simulink model "PhaseII_opalrt_NoProtection"  (Simulink 8.8)
settings: Solver=ode3  StartTime=0.0  StopTime=inf  FixedStep=Ts  RelTol=1e-5  EnableMultiTasking=on
PostLoadFcn:
  | %BESS ctrl
  | Kpf=0.005*3*12;
  | Kif=5*6;
  | 
  | Kpf1=0.005*3*12;
  | Kif1=5*6;
  | Kp_v=0.016*15*35;
  | Ki_v=12*25;
  | 
  | Kp_v1=0.016*15*35;
  | Ki_v1=12*25;
  | 
  | Vabc_B=12.47e3;
  | Vdc_ref=Vabc_B*2;
  | Kpwm=sqrt(2)*Vabc_B/Vdc_ref;
  | ZB=Vabc_B^2/1e6;
  | R=0.005*ZB;
  | Ibasefull=673/2*sqrt(2);
  | 
  | 
  | Ts_Control=1e-4;
  | ts=0.05;
  | delay=0.2;
  | offset=10e3;
  | t_plan=60;
  | t_monitor=.2;
  | t_mon=t_monitor;
  | scalingfactor=1;
  | x=0.5;
  | n=6;
  | %t_plan=1/15;
  | %t_monitor=10/900;
  | %t_mon=10/900;
  | 
  | %t_plan=1/5;
  | %t_monitor=10/300;
  | %t_mon=10/300;
  | %scalingfactor=1/300;
  | 
  | f0=60;
  | 
  | Pabc_B=1e6;
  | Iabc_B=Pabc_B*sqrt(2/3)/Vabc_B;  % pk value
  | Imax_1=2.5;
  | Ptrans_B=Pabc_B*200;
  | 
  | Vdc_ref=Vabc_B*2;
  | 
  | ZB=Vabc_B^2/Pabc_B;
  | L=0.1*ZB/2/pi/60;
  | R=0.1*ZB;
  | C=1/(4*pi^2*(2e3)^2*L);
  | 
  | LL=0.005*ZB/2/pi/60;
  | RR=0.005*ZB;
  | 
  | RC=0.02;
  | 
  | %%% Initial SOC %%%%
  | SOC_ini_BESS1=0.5;
  | ... (+223 lines)
InitFcn:
  | %BESS ctrl
  | Kpf=0.005*3*12;
  | Kif=5*6;
  | 
  | Kpf1=0.005*3*12;
  | Kif1=5*6;
  | Kp_v=0.016*15*35;
  | Ki_v=12*25;
  | 
  | Kp_v1=0.016*15*35;
  | Ki_v1=12*25;
  | 
  | Vabc_B=12.47e3;
  | Vdc_ref=Vabc_B*2;
  | Kpwm=sqrt(2)*Vabc_B/Vdc_ref;
  | ZB=Vabc_B^2/1e6;
  | R=0.005*ZB;
  | Ibasefull=673/2*sqrt(2);
  | 
  | 
  | Ts_Control=1e-4;
  | ts=0.05;
  | delay=0.2;
  | offset=10e3;
  | t_plan=60;
  | t_monitor=.2;
  | t_mon=t_monitor;
  | scalingfactor=1;
  | x=0.5;
  | n=6;
  | %t_plan=1/15;
  | %t_monitor=10/900;
  | %t_mon=10/900;
  | 
  | %t_plan=1/5;
  | %t_monitor=10/300;
  | %t_mon=10/300;
  | %scalingfactor=1/300;
  | 
  | f0=60;
  | 
  | Pabc_B=1e6;
  | Iabc_B=Pabc_B*sqrt(2/3)/Vabc_B;  % pk value
  | Imax_1=2.5;
  | Ptrans_B=Pabc_B*200;
  | 
  | Vdc_ref=Vabc_B*2;
  | 
  | ZB=Vabc_B^2/Pabc_B;
  | L=0.1*ZB/2/pi/60;
  | R=0.1*ZB;
  | C=1/(4*pi^2*(2e3)^2*L);
  | 
  | LL=0.005*ZB/2/pi/60;
  | RR=0.005*ZB;
  | 
  | RC=0.02;
  | 
  | %%% Initial SOC %%%%
  | SOC_ini_BESS1=0.5;
  | ... (+223 lines)
undefined symbols (not defined in the file): D1, Delta, DiscIntNeverNeededParam, Left, PG2ref, type, V
libraries: powerlib x220, powerlib_meascontrol x82, dspstat3 x54, dsparch4 x43, dspswit3 x24, simulink x19, simulink_extras x12, powerlib_extras x11, ssn_lib x7, artemis x6, rtlab x5, rtio_generic_dnp3 x5
(part 4 of 9)

== system PhaseII_opalrt_NoProtection/SM_System/PV Farm 2 MW1 ==
  Demux2 : Demux  Outputs=3
  Gain5 : Gain  Gain=Vdc_ref/2
  vsa : powerlib/Electrical Sources/Controlled Voltage Source  Initialize=on  Source_Type=AC  Amplitude=0  Phase=0  Frequency=0  Measurements=None
  vsb : powerlib/Electrical Sources/Controlled Voltage Source  Initialize=on  Source_Type=AC  Amplitude=0  Phase=0  Frequency=0  Measurements=None
  vsc : powerlib/Electrical Sources/Controlled Voltage Source  Initialize=on  Source_Type=AC  Amplitude=0  Phase=0  Frequency=0  Measurements=None
  A : PMIOPort  Tag=PMCPort  Port=1  Side=Right
  B : PMIOPort  Tag=PMCPort  Port=2  Side=Right
  C : PMIOPort  Tag=PMCPort  Port=3  Side=Right
  wires:
  Demux2/1 -> vsa/1
  Demux2/2 -> vsb/1
  Demux2/3 -> vsc/1
  [Vref_PV1] -> Gain5/1
  Gain5/1 -> Demux2/1
  connections:
  vsa/LConn1 -- vsc/LConn1 -- vsb/LConn1
  vsc/RConn1 -- C/RConn1
  B/RConn1 -- vsb/RConn1
  vsa/RConn1 -- A/RConn1

== system PhaseII_opalrt_NoProtection/SM_System/Subsystem ==
  In1 : Inport
  Fault : Subsystem
  Ground : powerlib/Elements/Ground  LConnTagsString=a
  Three-Phase Series RLC Branch5 : powerlib/Elements/Three-Phase Series RLC Branch  LConnTagsString=A|B|C  RConnTagsString=A|B|C  BranchType=RL  Resistance=1e-2  Inductance=1e-2  Capacitance=1e-4  Measurements=None
  a : PMIOPort  Port=1  Side=Left
  b : PMIOPort  Port=2  Side=Left
  c : PMIOPort  Port=3  Side=Left
  wires:
  In1/1 -> Fault/1(In7)
  connections:
  Ground/LConn1 -- Three-Phase Series RLC Branch5/LConn3 -- Three-Phase Series RLC Branch5/LConn2 -- Three-Phase Series RLC Branch5/LConn1
  Fault/RConn2 -- Three-Phase Series RLC Branch5/RConn2
  Fault/RConn3 -- Three-Phase Series RLC Branch5/RConn3
  Fault/RConn1 -- Three-Phase Series RLC Branch5/RConn1
  a/RConn1 -- Fault/LConn1
  b/RConn1 -- Fault/LConn2
  c/RConn1 -- Fault/LConn3

== system PhaseII_opalrt_NoProtection/SM_System/Subsystem1 ==
  In1 : Inport
  Fault : Subsystem
  Ground : powerlib/Elements/Ground  LConnTagsString=a
  Three-Phase Series RLC Branch5 : powerlib/Elements/Three-Phase Series RLC Branch  LConnTagsString=A|B|C  RConnTagsString=A|B|C  BranchType=RL  Resistance=1e-2  Inductance=1e-2  Capacitance=1e-4  Measurements=None
  a : PMIOPort  Port=1  Side=Left
  b : PMIOPort  Port=2  Side=Left
  c : PMIOPort  Port=3  Side=Left
  wires:
  In1/1 -> Fault/1(In7)
  connections:
  c/RConn1 -- Fault/LConn3
  b/RConn1 -- Fault/LConn2
  a/RConn1 -- Fault/LConn1
  Fault/RConn1 -- Three-Phase Series RLC Branch5/RConn1
  Fault/RConn3 -- Three-Phase Series RLC Branch5/RConn3
  Fault/RConn2 -- Three-Phase Series RLC Branch5/RConn2
  Three-Phase Series RLC Branch5/LConn1 -- Three-Phase Series RLC Branch5/LConn2 -- Three-Phase Series RLC Branch5/LConn3 -- Ground/LConn1

== system PhaseII_opalrt_NoProtection/SM_System/Subsystem2 ==
  In1 : Inport
  Fault : Subsystem
  Ground : powerlib/Elements/Ground  LConnTagsString=a
  Three-Phase Series RLC Branch5 : powerlib/Elements/Three-Phase Series RLC Branch  LConnTagsString=A|B|C  RConnTagsString=A|B|C  BranchType=RL  Resistance=1e-2  Inductance=1e-2  Capacitance=1e-4  Measurements=None
  a : PMIOPort  Port=1  Side=Left
  b : PMIOPort  Port=2  Side=Left
  c : PMIOPort  Port=3  Side=Left
  wires:
  In1/1 -> Fault/1(In7)
  connections:
  Ground/LConn1 -- Three-Phase Series RLC Branch5/LConn3 -- Three-Phase Series RLC Branch5/LConn2 -- Three-Phase Series RLC Branch5/LConn1
  Fault/RConn2 -- Three-Phase Series RLC Branch5/RConn2
  Fault/RConn3 -- Three-Phase Series RLC Branch5/RConn3
  Fault/RConn1 -- Three-Phase Series RLC Branch5/RConn1
  a/RConn1 -- Fault/LConn1
  b/RConn1 -- Fault/LConn2
  c/RConn1 -- Fault/LConn3

== system PhaseII_opalrt_NoProtection/SM_System/Subsystem3 ==
  In1 : Inport
  Fault : Subsystem
  Ground : powerlib/Elements/Ground  LConnTagsString=a
  Three-Phase Series RLC Branch5 : powerlib/Elements/Three-Phase Series RLC Branch  LConnTagsString=A|B|C  RConnTagsString=A|B|C  BranchType=RL  Resistance=1e-2  Inductance=1e-2  Capacitance=1e-4  Measurements=None
  a : PMIOPort  Port=1  Side=Left
  b : PMIOPort  Port=2  Side=Left
  c : PMIOPort  Port=3  Side=Left
  wires:
  In1/1 -> Fault/1(In7)
  connections:
  c/RConn1 -- Fault/LConn3
  b/RConn1 -- Fault/LConn2
  a/RConn1 -- Fault/LConn1
  Fault/RConn1 -- Three-Phase Series RLC Branch5/RConn1
  Fault/RConn3 -- Three-Phase Series RLC Branch5/RConn3
  Fault/RConn2 -- Three-Phase Series RLC Branch5/RConn2
  Three-Phase Series RLC Branch5/LConn1 -- Three-Phase Series RLC Branch5/LConn2 -- Three-Phase Series RLC Branch5/LConn3 -- Ground/LConn1

== system PhaseII_opalrt_NoProtection/SM_System/Subsystem4 ==
  In1 : Inport
  Fault : Subsystem
  Ground : powerlib/Elements/Ground  LConnTagsString=a
  Three-Phase Series RLC Branch5 : powerlib/Elements/Three-Phase Series RLC Branch  LConnTagsString=A|B|C  RConnTagsString=A|B|C  BranchType=RL  Resistance=1e-2  Inductance=1e-2  Capacitance=1e-4  Measurements=None
  a : PMIOPort  Port=1  Side=Left
  b : PMIOPort  Port=2  Side=Left
  c : PMIOPort  Port=3  Side=Left
  wires:
  In1/1 -> Fault/1(In7)
  connections:
  Ground/LConn1 -- Three-Phase Series RLC Branch5/LConn3 -- Three-Phase Series RLC Branch5/LConn1 -- Three-Phase Series RLC Branch5/LConn2
  Fault/RConn2 -- Three-Phase Series RLC Branch5/RConn2
  Fault/RConn3 -- Three-Phase Series RLC Branch5/RConn3
  Fault/RConn1 -- Three-Phase Series RLC Branch5/RConn1
  a/RConn1 -- Fault/LConn1
  b/RConn1 -- Fault/LConn2
  c/RConn1 -- Fault/LConn3

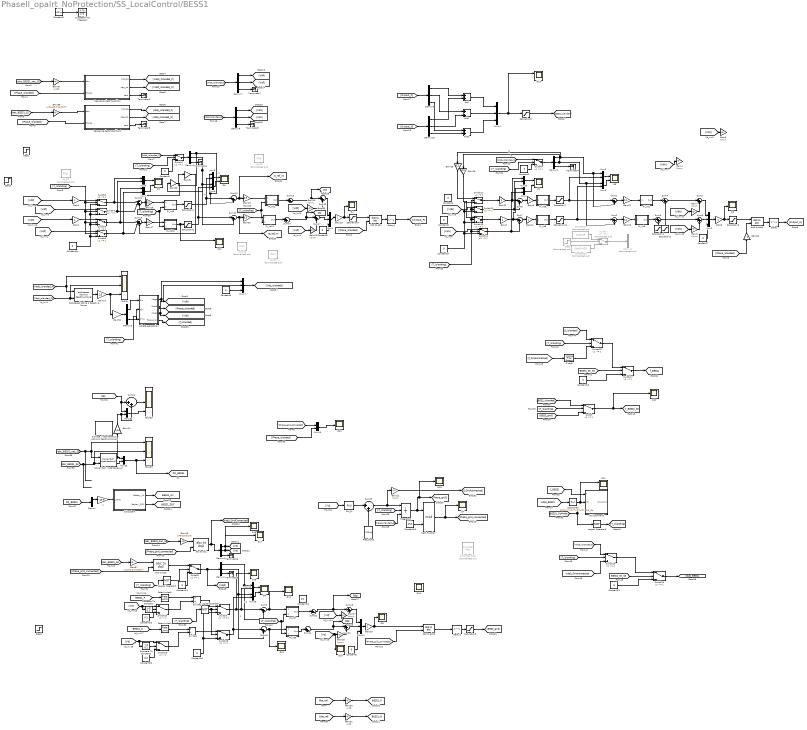
== system PhaseII_opalrt_NoProtection/SS_LocalControl/BESS1 ==
  "     1" : Gain  Gain=-1e-6
  2 kHz5 : dsparch4/Analog Filter Design  method=Butterworth  filttype=Lowpass  N=2  Wlo=2*pi*1  Whi=80  Rp=2  Rs=40
  2nd-Order Filter : powerlib_extras/Control  Blocks/2nd-Order Filter  Commented=on  FilterType=Lowpass  Fo=25  Zeta=0.707  Initialize=on  Vac_Init=[0 0 60]  Vdc_Init=377  PlotResponse=off  param1=[1 1000 0.5]
  3-phase  Instantaneous  Active & Reactive Power3 : powerlib_extras/Measurements/3-phase  Instantaneous  Active & Reactive Power
  Add : Sum
  Add1 : Sum
  Add2 : Sum
  Compare To Constant : simulink/Logic and Bit Operations/Compare To Constant  relop=>=  const=0.2  OutDataTypeStr=boolean
  Compare To Constant1 : simulink/Logic and Bit Operations/Compare To Constant  relop=>=  const=0.2  OutDataTypeStr=boolean
  Constant{1..2,4..11,13..14,17,21} (14 alike) : Constant  Value=0  SampleTime=-1
  Constant12 : Constant  Value=0.1  SampleTime=-1
  Constant15 : Constant  Value=2*pi
  Constant16 : Constant  Value=0.2  SampleTime=-1
  Constant18 : Constant  Commented=on  Value=[Kpf1 Kif1]  SampleTime=-1
  Constant19 : Constant  Commented=on  Value=[Kpf Kif]  SampleTime=-1
  Constant20 : Constant  Value=0.2  SampleTime=-1
  Constant3 : Constant  Value=120*pi
  D{1..2,5..6,9,15,22} (7 alike) : Scope  NumInputPorts=2
  D{3..4,7..8,10..14,16..20} (14 alike) : Scope
  D21 : Scope  NumInputPorts=3
  Delay : Delay  DelayLength=1  InitialCondition=0
  Delay1 : Delay  DelayLength=1  InitialCondition=0
  Delay2 : Delay  DelayLength=1  InitialCondition=0
  Demux : Demux  Outputs=2
  Demux1 : Demux  Commented=on  Outputs=2
  Demux{2,4..10} (8 alike) : Demux  Outputs=3
  Demux3 : Demux  Outputs=2
  Discrete-Time Integrator : DiscreteIntegrator  SampleTime=-1  ICPrevOutput=DiscIntNeverNeededParam  ICPrevScaledInput=DiscIntNeverNeededParam
  Divide1 : Product  Inputs=*/
  Divide2 : Product  Inputs=*/
  Freq_Const : Constant  Value=120*pi
  Gain{1..3,6,8,11,15,22,29} (9 alike) : Gain
  Gain{4..5,7,9..10,13,27..28} (8 alike) : Gain  Gain=Kpwm
  Gain12 : Gain  Gain=0.1
  Gain14 : Gain  Gain=2/3
  Gain{16..18,20} (4 alike) : Gain  Gain=0.5
  Gain19 : Gain  Gain=1/480/sqrt(2/3)
  Gain21 : Gain  Gain=1/2/pi
  Gain23 : Gain  Gain=0.1
  Gain24 : Gain  Gain=-1e-6
  Gain25 : Gain  Gain=0.2
  Gain26 : Gain  Gain=0.2
  Gain30 : Gain  Gain=-4.38
  Gain31 : Gain  Gain=-4.38
  Gain32 : Gain  Gain=0.228
  Gain33 : Gain  Gain=0.12
  Gain34 : Gain  Gain=0.12
  Gain36 : Gain  Gain=-1
  Gain37 : Gain  Gain=1/sqrt(2/3)/Ibasefull
  Gain38 : Gain  Gain=1/Ibasefull/sqrt(2/3)
  Gain57 : Gain  Gain=1/480
  ID&IQ : Scope  NumInputPorts=3
  ID&IQ1 : Scope  NumInputPorts=3
  ID&IQ2 : Scope  NumInputPorts=3
  Integrator1 : Integrator  ExternalReset=falling  InitialConditionSource=external  LimitOutput=on
  Logical Operator : Logic  Operator=NOT  Inputs=1  AllPortsSameDT=off  OutDataTypeStr=boolean
  Logical Operator1 : Logic  Operator=NOT  Inputs=1  AllPortsSameDT=off  OutDataTypeStr=boolean
  Logical Operator3 : Logic  Operator=NOT  AllPortsSameDT=off  OutDataTypeStr=boolean
  Math Function : Math  Operator=mod  SaturateOnIntegerOverflow=on
  Mux{1..2,11,14,17} (5 alike) : Mux  Inputs=3
  Mux{3..10,12..13,15..16,18} (13 alike) : Mux  Inputs=2
  PI_Vd1 : Subsystem
  PI_Vd10 : Subsystem
  PI_Vd11 : Subsystem
  PI_Vd2 : Subsystem
  PI_Vd3 : Subsystem
  PI_Vd5 : Subsystem
  PI_Vd6 : Subsystem
  PI_Vd7 : Subsystem
  PI_Vd8 : Subsystem
  PI_Vd9 : Subsystem
  PLL_PI : simulink/Continuous/PID Controller  Controller=PI  TimeDomain=Continuous-time  SampleTime=-1  IntegratorMethod=Forward Euler  FilterMethod=Forward Euler  Form=Parallel  UseFilter=on  ControllerParametersSource=internal  P=53*100  I=900*100  D=0  N=100  InitialConditionSource=internal  InitialConditionForIntegrator=0  InitialConditionForFilter=0  ExternalReset=none  ZeroCross=off  LimitOutput=on  UpperSaturationLimit=20  LowerSaturationLimit=-20  LinearizeAsGain=off  AntiWindupMode=clamping  Kb=1  TrackingMode=off  Kt=1  PParamMin=[]  PParamMax=[]  IParamMin=[]  IParamMax=[]  DParamMin=[]  DParamMax=[]  NParamMin=[]  NParamMax=[]  KbParamMin=[]  KbParamMax=[]  KtParamMin=[]  KtParamMax=[]  POutMin=[]  POutMax=[]  IOutMin=[]  IOutMax=[]  DOutMin=[]  DOutMax=[]  NOutMin=[]  NOutMax=[]  KbOutMin=[]  KbOutMax=[]  KtOutMin=[]  KtOutMax=[]  IntegratorOutMin=[]  IntegratorOutMax=[]  FilterOutMin=[]  FilterOutMax=[]  SumOutMin=[]  SumOutMax=[]  SumI1OutMin=[]  SumI1OutMax=[]  SumI2OutMin=[]  SumI2OutMax=[]  SumI3OutMin=[]  SumI3OutMax=[]  SumDOutMin=[]  SumDOutMax=[]  SaturationOutMin=[]  SaturationOutMax=[]  IntegratorContinuousStateAttributes=''  IntegratorStateMustResolveToSignalObject=off  IntegratorRTWStateStorageClass=Auto  FilterContinuousStateAttributes=''  FilterStateMustResolveToSignalObject=off  FilterRTWStateStorageClass=Auto  DifferentiatorICPrevScaledInput=0  DifferentiatorOutMin=[]  DifferentiatorOutMax=[]
  "Power (3ph, Instantaneous)" : powerlib_meascontrol/Measurements/Power (3ph, Instantaneous)
  Rate Limiter1 : RateLimiter  SampleTimeMode=inherited
  Rate Limiter2 : RateLimiter  SampleTimeMode=inherited
  SW Command : Subsystem
  Saturation1 : Saturate  UpperLimit=0.95  LowerLimit=-0.95
  Saturation10 : Saturate  UpperLimit=2  LowerLimit=-2  ZeroCross=off
  Saturation2 : Saturate  UpperLimit=0.95  LowerLimit=-0.95
  Saturation3 : Saturate  UpperLimit=1  LowerLimit=-1
  Saturation4 : Saturate  UpperLimit=4  LowerLimit=-4  ZeroCross=off
  Saturation5 : Saturate  UpperLimit=1.1  LowerLimit=-1.1  ZeroCross=off
  Saturation6 : Saturate  UpperLimit=6  LowerLimit=-6  ZeroCross=off
  Saturation7 : Saturate  UpperLimit=2  LowerLimit=-2  ZeroCross=off
  Saturation8 : Saturate  UpperLimit=1  LowerLimit=-1  ZeroCross=off
  Saturation9 : Saturate  UpperLimit=1  LowerLimit=-1  ZeroCross=off
  Sequence decomposition : Subsystem
  Sequence decomposition1 : Subsystem
  Step1 : Step  Time=0.5  SampleTime=0  ZeroCross=off
  Step2 : Step  Time=0  ZeroCross=off
  Step3 : Step  Time=0.5  SampleTime=0  ZeroCross=off
  Step6 : Step  Commented=on  Time=0.35  SampleTime=0
  Subsystem : Subsystem  mask{AH=100}
      mask prompts: AH "Capacity[Ah]"
      mask Display: image(imread(fullfile(matlabroot,'toolbox/physmod/powersys/DR/DRdemo/Battery.jpg')))
  Sum{1..2,6..7,9..11,18} (8 alike) : Sum  Inputs=|-+
  Sum{3,5,8,12,14,17,19,21..24} (11 alike) : Sum  Inputs=|++
  Sum13 : Sum  Inputs=|+-
  Sum15 : Sum  Inputs=|-++
  Sum16 : Sum  Inputs=|-+-
  Sum20 : Sum  Inputs=|+-
  Sum4 : Sum  Inputs=|+-
  Switch{,14,17..20} (6 alike) : Switch  Threshold=1
  Switch{1,3..6,8..9,11..13,15} (11 alike) : Switch  Threshold=1  ZeroCross=off
  Switch10 : Switch  Criteria=u2 > Threshold
  Switch16 : Switch  Criteria=u2 > Threshold
  Switch2 : Switch  Threshold=0.5  ZeroCross=off
  Switch7 : Switch  Commented=on  Threshold=1
  Terminator{1..8} (8 alike) : Terminator
  V_theta_generation : Subsystem
  Vd_PI10 : simulink/Continuous/PID Controller  Commented=on  Controller=PI  TimeDomain=Continuous-time  SampleTime=-1  IntegratorMethod=Trapezoidal  FilterMethod=Forward Euler  Form=Parallel  UseFilter=on  ControllerParametersSource=internal  P=Kpf1*5  I=Kif1*5  D=0  N=100  InitialConditionSource=internal  InitialConditionForIntegrator=0  InitialConditionForFilter=0  ExternalReset=none  LimitOutput=on  UpperSaturationLimit=1.2  LowerSaturationLimit=-1.2  LinearizeAsGain=off  AntiWindupMode=back-calculation  Kb=20  TrackingMode=off  Kt=1  PParamMin=[]  PParamMax=[]  IParamMin=[]  IParamMax=[]  DParamMin=[]  DParamMax=[]  NParamMin=[]  NParamMax=[]  KbParamMin=[]  KbParamMax=[]  KtParamMin=[]  KtParamMax=[]  POutMin=[]  POutMax=[]  IOutMin=[]  IOutMax=[]  DOutMin=[]  DOutMax=[]  NOutMin=[]  NOutMax=[]  KbOutMin=[]  KbOutMax=[]  KtOutMin=[]  KtOutMax=[]  IntegratorOutMin=[]  IntegratorOutMax=[]  FilterOutMin=[]  FilterOutMax=[]  SumOutMin=[]  SumOutMax=[]  SumI1OutMin=[]  SumI1OutMax=[]  SumI2OutMin=[]  SumI2OutMax=[]  SumI3OutMin=[]  SumI3OutMax=[]  SumDOutMin=[]  SumDOutMax=[]  SaturationOutMin=[]  SaturationOutMax=[]  IntegratorContinuousStateAttributes=''  IntegratorStateMustResolveToSignalObject=off  IntegratorRTWStateStorageClass=Auto  FilterContinuousStateAttributes=''  FilterStateMustResolveToSignalObject=off  FilterRTWStateStorageClass=Auto  DifferentiatorICPrevScaledInput=0  DifferentiatorOutMin=[]  DifferentiatorOutMax=[]
  Vd_PI2 : simulink/Continuous/PID Controller  Commented=on  Controller=PI  TimeDomain=Discrete-time  SampleTime=-1  IntegratorMethod=Forward Euler  FilterMethod=Forward Euler  Form=Parallel  UseFilter=on  ControllerParametersSource=internal  P=0.016*20  I=5*20  D=0  N=100  InitialConditionSource=internal  InitialConditionForIntegrator=0  InitialConditionForFilter=0  ExternalReset=none  LimitOutput=on  UpperSaturationLimit=0.5  LowerSaturationLimit=-0.5  LinearizeAsGain=off  AntiWindupMode=back-calculation  Kb=20  TrackingMode=off  Kt=1  PParamMin=[]  PParamMax=[]  IParamMin=[]  IParamMax=[]  DParamMin=[]  DParamMax=[]  NParamMin=[]  NParamMax=[]  KbParamMin=[]  KbParamMax=[]  KtParamMin=[]  KtParamMax=[]  POutMin=[]  POutMax=[]  IOutMin=[]  IOutMax=[]  DOutMin=[]  DOutMax=[]  NOutMin=[]  NOutMax=[]  KbOutMin=[]  KbOutMax=[]  KtOutMin=[]  KtOutMax=[]  IntegratorOutMin=[]  IntegratorOutMax=[]  FilterOutMin=[]  FilterOutMax=[]  SumOutMin=[]  SumOutMax=[]  SumI1OutMin=[]  SumI1OutMax=[]  SumI2OutMin=[]  SumI2OutMax=[]  SumI3OutMin=[]  SumI3OutMax=[]  SumDOutMin=[]  SumDOutMax=[]  SaturationOutMin=[]  SaturationOutMax=[]  IntegratorContinuousStateAttributes=''  IntegratorStateMustResolveToSignalObject=off  IntegratorRTWStateStorageClass=Auto  FilterContinuousStateAttributes=''  FilterStateMustResolveToSignalObject=off  FilterRTWStateStorageClass=Auto  DifferentiatorICPrevScaledInput=0  DifferentiatorOutMin=[]  DifferentiatorOutMax=[]
  Vd_PI6 : simulink/Continuous/PID Controller  Commented=on  Controller=PI  TimeDomain=Continuous-time  SampleTime=-1  IntegratorMethod=Forward Euler  FilterMethod=Forward Euler  Form=Parallel  UseFilter=on  ControllerParametersSource=internal  P=0.016*10  I=5*10  D=0  N=100  InitialConditionSource=internal  InitialConditionForIntegrator=0  InitialConditionForFilter=0  ExternalReset=none  LimitOutput=on  UpperSaturationLimit=3  LowerSaturationLimit=-3  LinearizeAsGain=off  AntiWindupMode=back-calculation  Kb=50  TrackingMode=off  Kt=1  PParamMin=[]  PParamMax=[]  IParamMin=[]  IParamMax=[]  DParamMin=[]  DParamMax=[]  NParamMin=[]  NParamMax=[]  KbParamMin=[]  KbParamMax=[]  KtParamMin=[]  KtParamMax=[]  POutMin=[]  POutMax=[]  IOutMin=[]  IOutMax=[]  DOutMin=[]  DOutMax=[]  NOutMin=[]  NOutMax=[]  KbOutMin=[]  KbOutMax=[]  KtOutMin=[]  KtOutMax=[]  IntegratorOutMin=[]  IntegratorOutMax=[]  FilterOutMin=[]  FilterOutMax=[]  SumOutMin=[]  SumOutMax=[]  SumI1OutMin=[]  SumI1OutMax=[]  SumI2OutMin=[]  SumI2OutMax=[]  SumI3OutMin=[]  SumI3OutMax=[]  SumDOutMin=[]  SumDOutMax=[]  SaturationOutMin=[]  SaturationOutMax=[]  IntegratorContinuousStateAttributes=''  IntegratorStateMustResolveToSignalObject=off  IntegratorRTWStateStorageClass=Auto  FilterContinuousStateAttributes=''  FilterStateMustResolveToSignalObject=off  FilterRTWStateStorageClass=Auto  DifferentiatorICPrevScaledInput=0  DifferentiatorOutMin=[]  DifferentiatorOutMax=[]
  Vd_PI8 : simulink/Continuous/PID Controller  Commented=on  Controller=PI  TimeDomain=Continuous-time  SampleTime=-1  IntegratorMethod=Trapezoidal  FilterMethod=Forward Euler  Form=Parallel  UseFilter=on  ControllerParametersSource=internal  P=Kpf1*5  I=Kif1*5  D=0  N=100  InitialConditionSource=internal  InitialConditionForIntegrator=0  InitialConditionForFilter=0  ExternalReset=none  LimitOutput=on  UpperSaturationLimit=1.2  LowerSaturationLimit=-1.2  LinearizeAsGain=off  AntiWindupMode=back-calculation  Kb=20  TrackingMode=off  Kt=1  PParamMin=[]  PParamMax=[]  IParamMin=[]  IParamMax=[]  DParamMin=[]  DParamMax=[]  NParamMin=[]  NParamMax=[]  KbParamMin=[]  KbParamMax=[]  KtParamMin=[]  KtParamMax=[]  POutMin=[]  POutMax=[]  IOutMin=[]  IOutMax=[]  DOutMin=[]  DOutMax=[]  NOutMin=[]  NOutMax=[]  KbOutMin=[]  KbOutMax=[]  KtOutMin=[]  KtOutMax=[]  IntegratorOutMin=[]  IntegratorOutMax=[]  FilterOutMin=[]  FilterOutMax=[]  SumOutMin=[]  SumOutMax=[]  SumI1OutMin=[]  SumI1OutMax=[]  SumI2OutMin=[]  SumI2OutMax=[]  SumI3OutMin=[]  SumI3OutMax=[]  SumDOutMin=[]  SumDOutMax=[]  SaturationOutMin=[]  SaturationOutMax=[]  IntegratorContinuousStateAttributes=''  IntegratorStateMustResolveToSignalObject=off  IntegratorRTWStateStorageClass=Auto  FilterContinuousStateAttributes=''  FilterStateMustResolveToSignalObject=off  FilterRTWStateStorageClass=Auto  DifferentiatorICPrevScaledInput=0  DifferentiatorOutMin=[]  DifferentiatorOutMax=[]
  abc to dq0 : powerlib_meascontrol/Transformations/abc to dq0  Alignment=90 degrees behind phase A axis
  abc to dq1 : powerlib_meascontrol/Transformations/abc to dq0  Alignment=90 degrees behind phase A axis
  dq0 to abc : powerlib_meascontrol/Transformations/dq0 to abc  Alignment=90 degrees behind phase A axis
  dq0 to abc1 : powerlib_meascontrol/Transformations/dq0 to abc  Alignment=90 degrees behind phase A axis
  dq0 to abc2 : powerlib_meascontrol/Transformations/dq0 to abc  Alignment=90 degrees behind phase A axis
  dq0-based Active & Reactive Power : powerlib_extras/Measurements/dq0-based Active & Reactive Power
  dq2alpha3 : Fcn  Expr=sqrt(u(1)*u(1)+u(2)*u(2))
  tag scope: BESS1_Ah=global, BESS1_P=global, BESS1_Q=global, BESS1_SOC=global, Ddg=global, Ddi=global, Dqg=global, Dqi=global, Id_ref_ini=global, Iq_ref_ini=global, PQ_BESS1=global, Phase_grid1=global, V_BESS1_SS=global, Vdq0_BESS1=global, f_BESS1=global
  wires:
  Mux9/1 -> D2/1
  Demux5/1 -> Gain34/1, Sum10/2, Mux6/1  "Id"
  Constant5/1 -> Mux1/3
  Sum14/1 -> [Dqi], Sum17/1
  Gain17/1 -> PI_Vd10/1(Error)
  Gain16/1 -> PI_Vd8/1(Error)
  Sum15/1 -> Gain16/1
  Demux5/3 -> Terminator1/1
  [VqP] -> Gain13/1
  Mux8/1 -> D6/2
  Mux1/1 -> Gain15/1
  Sum12/1 -> Mux1/1
  [Vq0] -> Gain1/1
  Gain20/1 -> PI_Vd11/1(Error)
  Sum13/1 -> [Ddi], Sum12/1
  PI_Vd11/1(Out) -> Sum14/1
  Gain15/1 -> Saturation9/1, D4/1
  [VdP] -> Gain10/1
  Sum16/1 -> Gain17/1
  Demux5/2 -> Gain33/1, Mux8/1, Sum11/2  "Iq"
  Mux7/1 -> D2/2
  Mux6/1 -> D6/1
  Sum10/1 -> [Id_ref_ini], Gain18/1
  Sum11/1 -> [Iq_ref_ini], Gain20/1
  [Vd0] -> Gain2/1
  Sum17/1 -> Mux1/2
  [Vabc_BESS1_sec_SS] -> Gain57/1
  [Iabc_BESS1_SS] -> Gain38/1
  Constant3/1 -> Discrete-Time Integrator/1
  [Phase_islanded] -> Sequence decomposition/2(Phase)
  [Phase_islanded] -> Sequence decomposition1/2(Phase)
  Sequence decomposition/1(Pos_dq) -> [Vdq0_islanded_P]
  Sequence decomposition/2(Neg_dq) -> [Vdq0_islanded_N]
  Sequence decomposition/3(zero) -> Terminator2/1
  Sequence decomposition1/1(Pos_dq) -> [Idq0_islanded_P]
  Sequence decomposition1/2(Neg_dq) -> [Idq0_islanded_N]
  Sequence decomposition1/3(zero) -> Terminator3/1
  Saturation9/1 -> dq0 to abc/1
  [Phase_islanded] -> dq0 to abc/2
  Constant7/1 -> Mux2/3
  Sum7/1 -> Gain11/1
  Mux3/1 -> D5/1
  Switch14/1 -> Sum7/2, Mux4/2
  Mux4/1 -> D1/2
  Sum1/1 -> Gain12/1
  Gain11/1 -> PI_Vd6/1(Error)
  Sum5/1 -> Sum8/1
  Mux10/1 -> D1/1
  Demux2/3 -> Terminator4/1
  Gain22/1 -> Mux10/1, Sum6/1
  Saturation1/1 -> Sum5/2
  Sum2/1 -> Gain23/1
  Gain12/1 -> PI_Vd2/1(Error)
  Sum6/1 -> Gain8/1
  PI_Vd3/1(Out) -> Sum5/1
  Sum4/1 -> Sum3/1
  Saturation2/1 -> Sum4/2
  Gain6/1 -> D3/1, Saturation3/1
  Switch12/1 -> Mux10/2, Sum6/2
  Gain3/1 -> Mux4/1, Sum7/1
  Mux5/1 -> D5/2
  [VqN] -> Gain5/1
  PI_Vd2/1(Out) -> Sum4/1
  [VdN] -> Gain4/1
  [Phase_islanded] -> Gain36/1
  Mux2/1 -> Gain6/1
  Saturation3/1 -> dq0 to abc1/1
  [Vdq0_islanded_P] -> Demux7/1
  Demux7/1 -> [VdP]
  Demux7/2 -> [VqP]
  Demux7/3 -> Terminator7/1
  Demux8/1 -> [VdN]
  Demux8/3 -> Terminator8/1
  Demux8/2 -> [VqN]
  [Vdq0_islanded_N] -> Demux8/1
  Gain36/1 -> dq0 to abc1/2
  [Output_P] -> Demux9/1
  [Output_N] -> Demux10/1
  Demux9/1 -> Add/1
  Demux10/1 -> Add/2
  Demux9/2 -> Add1/1
  Demux10/2 -> Add1/2
  Demux9/3 -> Add2/1
  Demux10/3 -> Add2/2
  Add1/1 -> Mux14/2
  Add/1 -> Mux14/1
  Add2/1 -> Mux14/3
  Mux14/1 -> D15/1, Saturation5/1
  [T_islanding] -> Switch/2
  [BESS_islanded] -> Switch/1
  [BESS_grid] -> Switch/3
  Gain2/1 -> Switch3/1
  [VdP] -> Switch4/1
  Gain1/1 -> Switch5/1
  [VqP] -> Switch6/1
  Constant14/1 -> Switch6/3, Switch5/3, Switch4/3, Switch3/3
  Switch3/1 -> Mux9/1, Sum15/1
  Switch4/1 -> Mux9/2, Sum15/2
  Switch5/1 -> Mux7/1, Sum16/1
  Switch6/1 -> Mux7/2, Sum16/2
  PI_Vd8/1(Out) -> Saturation4/1
  Switch11/1 -> Gain22/1
  [VqN] -> Switch14/1
  Switch13/1 -> Gain3/1
  [VdN] -> Switch12/1
  Constant17/1 -> Switch14/3, Switch13/3, Switch12/3, Switch11/3
  [T_islanding] -> Switch14/2, Switch13/2, Switch12/2, Switch11/2
  Demux2/1 -> Gain25/1, Sum1/2, Mux3/1  "Id"
  Demux2/2 -> Gain26/1, Sum2/2, Mux5/1  "Iq"
  Gain38/1 -> Sequence decomposition1/1(abc)
  Gain57/1 -> Sequence decomposition/1(abc)
  Gain23/1 -> PI_Vd3/1(Error)
  Sum3/1 -> Mux2/1
  Sum8/1 -> Mux2/2
  Step6/1 -> Switch7/2
  Constant18/1 -> Switch7/3
  Switch7/1 -> Demux1/1
  Constant19/1 -> Switch7/1
  [VdN] -> Gain7/1
  [VqN] -> Gain9/1
  Gain10/1 -> Sum12/2
  Gain13/1 -> Sum17/2
  Gain7/1 -> Sum3/2
  Gain9/1 -> Sum8/2
  Saturation5/1 -> [BESS_islanded]
  Gain8/1 -> PI_Vd5/1(Error)
  [Vdq0_islanded_P] -> ID&IQ/1, dq0-based Active & Reactive Power/1
  dq0-based Active & Reactive Power/1 -> Gain14/1
  Gain14/1 -> Gain32/1, ID&IQ/3
  [Idq0_islanded_P] -> ID&IQ/2, dq0-based Active & Reactive Power/2
  Demux3/1 -> V_theta_generation/1(Pin)
  Demux3/2 -> V_theta_generation/2(Qin)
  V_theta_generation/2(theta) -> [Phase_islanded]
  Delay1/1 -> [Output_P]
  dq0 to abc1/1 -> Delay/1
  dq0 to abc/1 -> Delay1/1
  V_theta_generation/1(Magd) -> [Vd0], Mux17/1
  V_theta_generation/3(Magq) -> [Vq0], Mux17/2
  Demux6/2 -> D13/1, [Vq]
  dq0 to abc2/1 -> Delay2/1
  Delay2/1 -> Saturation8/1
  Gain37/1 -> abc to dq0/1
  Demux4/3 -> Terminator5/1
  Sum9/1 -> PI_Vd7/1(Error), D11/1
  Switch8/1 -> [Idq0], Demux4/1
  Freq_Const/1 -> Sum23/2
  [Phase_grid_connected] -> abc to dq1/2
  [Phase_grid_connected] -> abc to dq0/2
  Demux6/3 -> Terminator6/1
  Sum18/1 -> PI_Vd9/1(Error), D12/1
  Constant8/1 -> Mux11/3
  Mux13/1 -> D9/2
  PI_Vd9/1(Out) -> Sum21/1
  Sum21/1 -> [Dqg], Sum22/1
  Sum22/1 -> Mux11/2
  Mux11/1 -> Gain29/1
  [Vq] -> PLL_PI/1
  PI_Vd7/1(Out) -> Sum20/1
  PLL_PI/1 -> Sum23/1
  [Iabc_BESS1_SS] -> Gain37/1
  [Vd] -> Gain27/1
  abc to dq0/1 -> Switch8/1
  Switch2/1 -> D18/1, Mux12/2, Sum9/1
  Mux12/1 -> D9/1
  Constant11/1 -> Switch8/3
  Demux4/1 -> Mux12/1, Sum9/2  "Id"
  [Phase_grid_connected] -> dq0 to abc2/2
  abc to dq1/1 -> [Vdq0_GridConnected], Demux6/1
  Demux6/1 -> D17/1, [Vd]
  Demux4/2 -> Mux13/1, Sum18/2  "Iq"
  Sum20/1 -> [Ddg], Sum19/1
  Gain29/1 -> dq0 to abc2/1, D8/1
  [Vq] -> D16/1, Gain28/1
  Sum19/1 -> Mux11/1
  Constant15/1 -> Math Function/2
  [Vabc_BESS1_sec_SS] -> Gain19/1
  Gain19/1 -> abc to dq1/1
  Math Function/1 -> D7/1, [Phase_grid_connected]
  Saturation8/1 -> [BESS_grid]
  Switch1/1 -> Demux5/1
  [Idq0_islanded_P] -> Switch1/1
  Constant1/1 -> Switch1/3
  Switch9/1 -> Demux2/1
  [Idq0_islanded_N] -> Switch9/1
  [T_islanding] -> Switch9/2
  Constant2/1 -> Switch9/3
  Saturation4/1 -> Sum10/1, Mux6/2
  Saturation6/1 -> Sum11/1, Mux8/2
  PI_Vd5/1(Out) -> Saturation7/1
  PI_Vd6/1(Out) -> Saturation10/1
  Saturation7/1 -> Sum1/1, Mux3/2
  Saturation10/1 -> Sum2/1, Mux5/2
  Constant16/1 -> Switch10/3
  Compare To Constant/1 -> Switch10/2
  [Vd] -> Compare To Constant/1, Switch10/1
  Switch10/1 -> Divide1/2
  [BESS1_P] -> Rate Limiter2/1
  Rate Limiter2/1 -> Divide1/1
  Divide1/1 -> Switch2/1
  [BESS1_Q] -> Rate Limiter1/1
  Divide2/1 -> Switch15/1
  Switch15/1 -> Sum18/1, Mux13/2
  Rate Limiter1/1 -> Divide2/1
  Compare To Constant1/1 -> Switch16/2
  [Vd] -> Compare To Constant1/1, Switch16/1
  Constant20/1 -> Switch16/3
  Switch16/1 -> Divide2/2
  Constant10/1 -> Switch15/3, Switch2/3
  [T_islanding] -> Switch3/2, Switch4/2, Switch5/2, Switch6/2
  [T_islanding] -> Switch1/2
  Gain27/1 -> Sum19/2
  Gain28/1 -> Sum22/2
  [Phase_grid_connected] -> Mux15/1
  [Phase_islanded] -> Mux15/2
  Mux15/1 -> D20/1
  Integrator1/1 -> D19/1, [Phase_grid1], Math Function/1
  [T_islanding] -> Integrator1/2
  [Phase_islanded_ref] -> Integrator1/3
  Logical Operator/1 -> Switch15/2, Switch2/2
  [T_islanding] -> Logical Operator/1
  [T_islanding] -> Logical Operator1/1
  Logical Operator1/1 -> Switch8/2
  Gain18/1 -> PI_Vd1/1(Error)
  PI_Vd1/1(Out) -> Sum13/1
  [f_BESS1] -> SW Command/1(f)
  [Vdq0_BESS1] -> dq2alpha3/1
  dq2alpha3/1 -> D21/1, SW Command/2(Vd)
  [BESS1_OpMode] -> SW Command/3(SW_Ctr), Logical Operator3/1
  Sum23/1 -> Gain21/1, Integrator1/1
  [Vabc_BESS1_sec_SS] -> "Power (3ph, Instantaneous)"/1, ID&IQ1/1
  [Iabc_BESS1_SS] -> "Power (3ph, Instantaneous)"/2, ID&IQ1/2
  Mux16/1 -> [PQ_BESS1], ID&IQ1/3
  "     1"/1 -> Subsystem/1(I_RMS)
  Subsystem/2(Battery_SOC) -> [BESS1_SOC]
  Subsystem/1(Battery_Ah) -> [BESS1_Ah]
  Demux/1 -> "     1"/1
  [PQ_BESS1] -> Demux/1
  PI_Vd10/1(Out) -> D22/1, Saturation6/1
  [T_islanding] -> PI_Vd10/2(T_islanding), PI_Vd8/2(T_islanding)
  [T_islanding] -> PI_Vd11/2(T_islanding), PI_Vd1/2(T_islanding)
  [T_islanding] -> PI_Vd9/2(T_islanding), PI_Vd7/2(T_islanding)
  Logical Operator3/1 -> [T_islanding]
  "Power (3ph, Instantaneous)"/2 -> Mux16/2
  [T_islanding] -> V_theta_generation/3(Pin1)
  Gain21/1 -> [f_Gridconnected]
  [BESS1_En_SS] -> Switch17/2
  [T_islanding] -> Switch18/2
  V_theta_generation/4(frequency) -> [f_islanded]
  [f_islanded] -> Switch18/1
  [f_Gridconnected] -> 2 kHz5/1
  [T_islanding] -> Switch19/2
  [Vdq0_islanded_P] -> Switch19/1
  [Vdq0_Gridconnected] -> Switch19/3
  Constant13/1 -> Switch17/3
  Mux17/1 -> [Vdq_islanded]
  Constant9/1 -> Mux17/3
  Switch/1 -> D10/1, [V_BESS1_SS]
  Switch17/1 -> [f_BESS1]
  Switch18/1 -> Switch17/1
  [BESS1_En_SS] -> Switch20/2
  Constant21/1 -> Switch20/3
  Switch20/1 -> [Vdq0_BESS1]
  Switch19/1 -> Switch20/1
  [Pba_ref] -> Gain30/1
  [Qba_ref] -> Gain31/1
  [Pe2] -> Sum24/1, Mux18/1
  "Power (3ph, Instantaneous)"/1 -> Mux16/1, Gain24/1
  Mux18/1 -> ID&IQ2/3
  Gain24/1 -> Sum24/2, Mux18/2
  Sum24/1 -> ID&IQ2/2
  Delay/1 -> [Output_N]
  Gain25/1 -> Switch11/1
  Gain26/1 -> Switch13/1
  Gain30/1 -> [BESS1_P]
  Gain31/1 -> [BESS1_Q]
  Gain32/1 -> Demux3/1
  Gain33/1 -> Sum15/3
  Gain34/1 -> Sum16/3
  2 kHz5/1 -> Switch18/3
